simulink model "test_sensor_fusion2"  (Simulink 7.6)
settings: Solver=ode45  StartTime=0.0  StopTime=2500.0  RelTol=1e-3
libraries: simulink x12
settings Model: Creator=jporter  LastModifiedBy=jporter

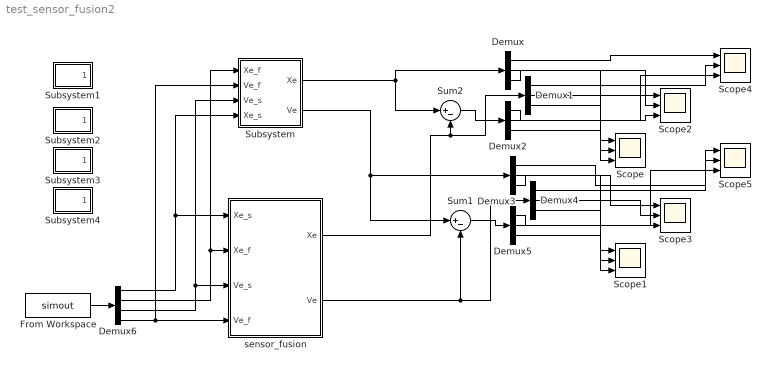
== system test_sensor_fusion2 ==
  Demux{,1..5} (6 alike) : Demux  Outputs=3
  Demux6 : Demux
  From Workspace : FromWorkspace  VariableName=simout  SampleTime=0.02  Interpolate=off  OutputAfterFinalValue=Holding final value
  Scope{,1..5} (6 alike) : Scope  NumInputPorts=3
      Scope settings: YMin=-5~-5~-5  YMax=5~5~5
      Scope1 settings: YMin=-5~-5~-5  YMax=5~5~5
      Scope2 settings: YMin=-5~-5~-5  YMax=5~5~5  SaveName=ScopeData2
      Scope3 settings: YMin=-5~-5~-5  YMax=5~5~5  SaveName=ScopeData3
      Scope4 settings: YMin=-5~-5~-5  YMax=5~5~5  SaveName=ScopeData4
      Scope5 settings: YMin=-5~-5~-5  YMax=5~5~5  SaveName=ScopeData5
  Subsystem : Subsystem
  Subsystem1 : Subsystem
  Subsystem2 : Subsystem
  Subsystem3 : Subsystem
  Subsystem4 : Subsystem
  Sum1 : Sum  Inputs=|+-
  Sum2 : Sum  Inputs=|+-
  sensor_fusion : Stateflow chart  TreatAsAtomicUnit=on
  wires:
  Subsystem/1(Xe) -> Sum2/1, Demux/1
  Subsystem/2(Ve) -> Sum1/1, Demux3/1
  sensor_fusion/2(Ve) -> Sum1/2, Demux4/1
  sensor_fusion/1(Xe) -> Sum2/2, Demux1/1
  Sum2/1 -> Demux2/1
  Sum1/1 -> Demux5/1
  Demux/3 -> Scope/1
  Demux1/3 -> Scope/2
  Demux2/3 -> Scope/3
  Demux3/3 -> Scope1/1
  Demux4/3 -> Scope1/2
  Demux5/3 -> Scope1/3
  From Workspace/1 -> Demux6/1
  Demux6/1 -> Subsystem/4(Xe_s), sensor_fusion/1(Xe_s)
  Demux6/2 -> Subsystem/1(Xe_f), sensor_fusion/2(Xe_f)
  Demux6/3 -> Subsystem/3(Ve_s), sensor_fusion/3(Ve_s)
  Demux6/4 -> Subsystem/2(Ve_f), sensor_fusion/4(Ve_f)
  Demux2/2 -> Scope2/3
  Demux1/2 -> Scope2/2
  Demux/2 -> Scope2/1
  Demux/1 -> Scope4/1
  Demux1/1 -> Scope4/2
  Demux2/1 -> Scope4/3
  Demux3/1 -> Scope5/1
  Demux4/1 -> Scope5/2
  Demux5/1 -> Scope5/3
  Demux3/2 -> Scope3/1
  Demux4/2 -> Scope3/2
  Demux5/2 -> Scope3/3

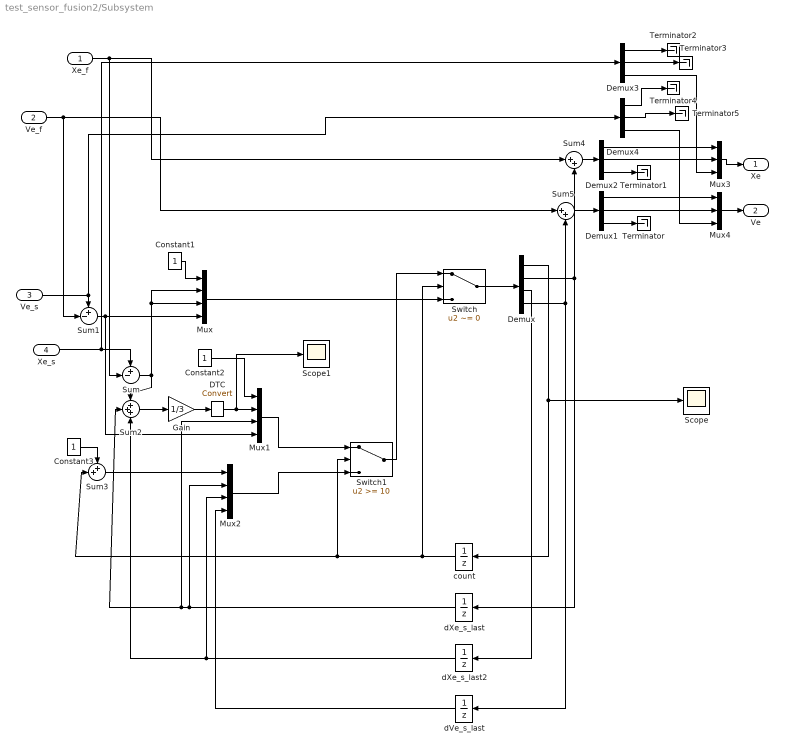
== system test_sensor_fusion2/Subsystem ==
  Xe_f : Inport
  Ve_f : Inport  Port=2
  Ve_s : Inport  Port=3
  Xe_s : Inport  Port=4
  Constant1 : Constant
  Constant2 : Constant
  Constant3 : Constant
  DTC : DataTypeConversion
  Demux : Demux  Outputs=[1 3 3 3]
  Demux{1..4} (4 alike) : Demux  Outputs=3
  Gain : Gain  Gain=1/3
  Mux : Mux  Inputs=[1 3 3 3]
  Mux1 : Mux  Inputs=[1 3 3 3]
  Mux2 : Mux  Inputs=[1 3 3 3]
  Mux3 : Mux  Inputs=3
  Mux4 : Mux  Inputs=3
  Scope : Scope
      settings: YMin=0  YMax=80  SaveName=ScopeData6
  Scope1 : Scope
      settings: YMin=0  YMax=80  SaveName=ScopeData7
  Sum : Sum  Inputs=+-|
  Sum1 : Sum  Inputs=+-|
  Sum2 : Sum  Inputs=+++
  Sum3 : Sum  Inputs=++|
  Sum4 : Sum  Inputs=|++
  Sum5 : Sum  Inputs=|++
  Switch : Switch  Criteria=u2 ~= 0
  Switch1 : Switch  Threshold=10
  Terminator{,1..5} (6 alike) : Terminator
  count : UnitDelay  SampleTime=-1
  dVe_s_last : UnitDelay  SampleTime=-1
  dXe_s_last : UnitDelay  SampleTime=-1
  dXe_s_last2 : UnitDelay  SampleTime=-1
  Xe : Outport
  Ve : Outport  Port=2
  wires:
  Xe_f/1 -> Sum/2, Sum4/1
  Ve_f/1 -> Sum1/2, Sum5/1
  count/1 -> Switch/2, Switch1/2, Sum3/2
  Switch1/1 -> Switch/1
  Mux/1 -> Switch/3
  Constant1/1 -> Mux/1
  Sum/1 -> Mux/2, Mux/3, Sum2/1
  Demux/1 -> count/1, Scope/1
  Demux/2 -> dXe_s_last/1, Sum4/2
  Demux/4 -> Sum5/2, dVe_s_last/1
  Sum1/1 -> Mux/4, Mux1/4
  Switch/1 -> Demux/1
  Mux1/1 -> Switch1/1
  Mux2/1 -> Switch1/3
  Constant2/1 -> Mux1/1
  dXe_s_last/1 -> Sum2/2, Mux1/3, Mux2/2
  dXe_s_last2/1 -> Mux2/3, Sum2/3
  Constant3/1 -> Sum3/1
  Sum3/1 -> Mux2/1
  dVe_s_last/1 -> Mux2/4
  Sum4/1 -> Demux2/1
  Sum5/1 -> Demux1/1
  Demux3/3 -> Mux3/3
  Demux4/3 -> Mux4/3
  Demux2/1 -> Mux3/1
  Demux2/2 -> Mux3/2
  Demux1/1 -> Mux4/1
  Demux1/2 -> Mux4/2
  Demux1/3 -> Terminator/1
  Demux2/3 -> Terminator1/1
  Mux3/1 -> Xe/1
  Mux4/1 -> Ve/1
  Ve_s/1 -> Sum1/1, Demux4/1
  Xe_s/1 -> Sum/1, Demux3/1
  Demux/3 -> dXe_s_last2/1
  Demux3/1 -> Terminator2/1
  Demux3/2 -> Terminator3/1
  Demux4/1 -> Terminator4/1
  Demux4/2 -> Terminator5/1
  Gain/1 -> DTC/1
  Sum2/1 -> Gain/1
  DTC/1 -> Mux1/2, Scope1/1

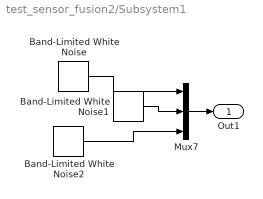
== system test_sensor_fusion2/Subsystem1 ==
  Band-Limited White Noise : simulink/Sources/Band-Limited White Noise  SystemSampleTime=-1  Cov=0.5  Ts=0.01  seed=[23341]
  Band-Limited White Noise1 : simulink/Sources/Band-Limited White Noise  SystemSampleTime=-1  Cov=0.5  Ts=0.01  seed=[23341]
  Band-Limited White Noise2 : simulink/Sources/Band-Limited White Noise  SystemSampleTime=-1  Cov=0.5  Ts=0.01  seed=[23341]
  Mux7 : Mux  Inputs=3
  Out1 : Outport
  wires:
  Band-Limited White Noise/1 -> Mux7/1
  Band-Limited White Noise1/1 -> Mux7/2
  Band-Limited White Noise2/1 -> Mux7/3
  Mux7/1 -> Out1/1

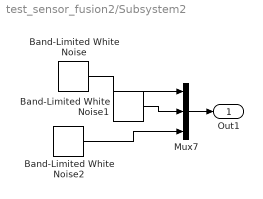
== system test_sensor_fusion2/Subsystem2 ==
  Band-Limited White Noise : simulink/Sources/Band-Limited White Noise  SystemSampleTime=-1  Cov=0.5  Ts=0.01  seed=[23341]
  Band-Limited White Noise1 : simulink/Sources/Band-Limited White Noise  SystemSampleTime=-1  Cov=0.5  Ts=0.01  seed=[23341]
  Band-Limited White Noise2 : simulink/Sources/Band-Limited White Noise  SystemSampleTime=-1  Cov=0.5  Ts=0.01  seed=[23341]
  Mux7 : Mux  Inputs=3
  Out1 : Outport
  wires:
  Band-Limited White Noise/1 -> Mux7/1
  Band-Limited White Noise1/1 -> Mux7/2
  Band-Limited White Noise2/1 -> Mux7/3
  Mux7/1 -> Out1/1

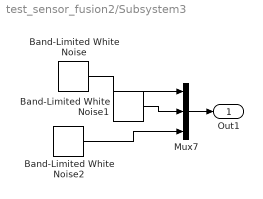
== system test_sensor_fusion2/Subsystem3 ==
  Band-Limited White Noise : simulink/Sources/Band-Limited White Noise  SystemSampleTime=-1  Cov=0.5  Ts=0.01  seed=[23341]
  Band-Limited White Noise1 : simulink/Sources/Band-Limited White Noise  SystemSampleTime=-1  Cov=0.5  Ts=0.01  seed=[23341]
  Band-Limited White Noise2 : simulink/Sources/Band-Limited White Noise  SystemSampleTime=-1  Cov=0.5  Ts=0.01  seed=[23341]
  Mux7 : Mux  Inputs=3
  Out1 : Outport
  wires:
  Band-Limited White Noise/1 -> Mux7/1
  Band-Limited White Noise1/1 -> Mux7/2
  Band-Limited White Noise2/1 -> Mux7/3
  Mux7/1 -> Out1/1

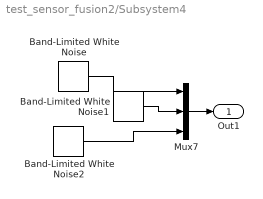
== system test_sensor_fusion2/Subsystem4 ==
  Band-Limited White Noise : simulink/Sources/Band-Limited White Noise  SystemSampleTime=-1  Cov=0.5  Ts=0.01  seed=[23341]
  Band-Limited White Noise1 : simulink/Sources/Band-Limited White Noise  SystemSampleTime=-1  Cov=0.5  Ts=0.01  seed=[23341]
  Band-Limited White Noise2 : simulink/Sources/Band-Limited White Noise  SystemSampleTime=-1  Cov=0.5  Ts=0.01  seed=[23341]
  Mux7 : Mux  Inputs=3
  Out1 : Outport
  wires:
  Band-Limited White Noise/1 -> Mux7/1
  Band-Limited White Noise1/1 -> Mux7/2
  Band-Limited White Noise2/1 -> Mux7/3
  Mux7/1 -> Out1/1

== matlab function sensor_fusion ==
  data: Xe_s input double; Xe output double; Xe_f input double; Ve_s input double; Ve_f input double; Ve output double
function [Xe,Ve] = fcn(Xe_s, Xe_f, Ve_s, Ve_f)
%Fuse the gps measurements Xe_s and Ve_s with the
%faster inertial sensor measurements Xe_f, Ve_f
%N.B. the height is updated by a fast pressure sensor so we always
%pass through the z-component of Xe_s and Ve_s
persistent count;
persistent dXe_s_last;
persistent dVe_s_last;
persistent dXe_s_last_2;
if isempty(count)
    count =  10;
    dXe_s_last = Xe_s-Xe_f;
    dXe_s_last_2 = dXe_s_last;
    dVe_s_last = Ve_s-Ve_f;
    dXe_s_last(3)=0;
    dVe_s_last(3)=0;
end
if count == 10
    count = 1; 
    temp = ((Xe_s(1:2)-Xe_f(1:2)) + dXe_s_last(1:2) + dXe_s_last_2(1:2))/3;
    dXe_s_last_2 = dXe_s_last;
    dXe_s_last(1:2) = temp;
    dVe_s_last(1:2) = Ve_s(1:2)-Ve_f(1:2);
else
    count = count + 1;
end
Xe = Xe_f + dXe_s_last;
Ve = Ve_f + dVe_s_last;
Xe(3) = Xe_s(3);
Ve(3) = Ve_s(3);
